simulink model "pid_pd_sim_2"  (R2016b)
settings: Solver=VariableStepAuto  StartTime=0.0  StopTime=100.0  FixedStep=1e-3  RelTol=1e3
values from neighbouring files (symbols this model uses):
  K_DG = part_vec(5)    [pso_tuning.m]
  K_filterG = 1/200    (= 0.005)    [pso_tuning.m]
undefined symbols (not defined in the file or in its folder): A_butter, B_butter, C_butter, D_butter, param, system
libraries: simulink x5
settings Model: Creator=nicol  LastModifiedBy=Fritz

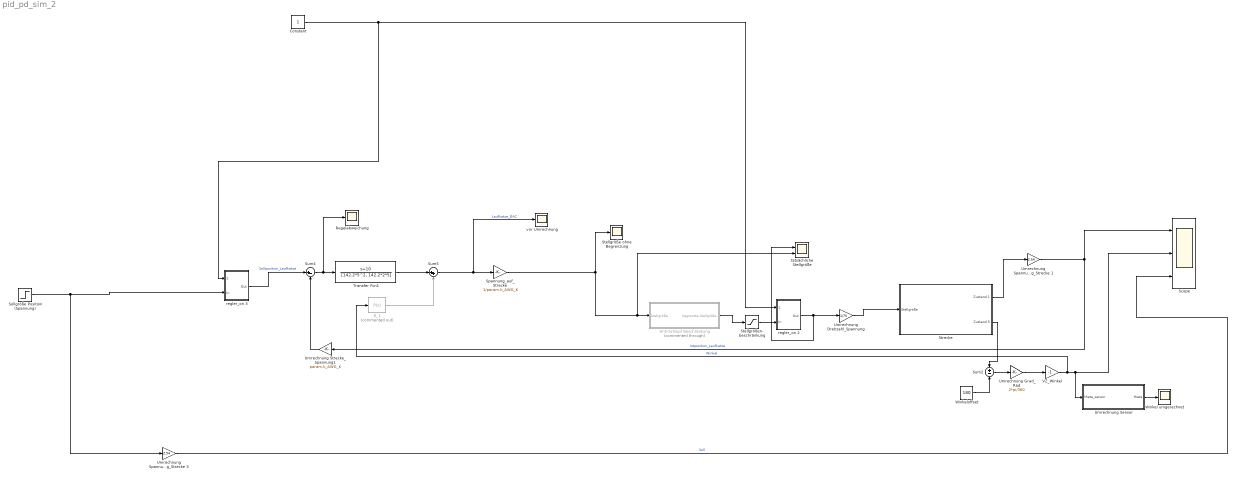
== system pid_pd_sim_2 ==
  Anti-Schlupf Beschränkung : Subsystem  Commented=through
  Constant : Constant
  R_1 : simulink/Continuous/PID Controller  Commented=on  Controller=P  TimeDomain=Continuous-time  SampleTime=-1  IntegratorMethod=Forward Euler  FilterMethod=Forward Euler  Form=Parallel  UseFilter=on  ControllerParametersSource=internal  P=0.1  I=0  D=K_DG  N=1/K_filterG  InitialConditionSource=internal  InitialConditionForIntegrator=0  InitialConditionForFilter=0  ExternalReset=none  LimitOutput=off  UpperSaturationLimit=inf  LowerSaturationLimit=-inf  LinearizeAsGain=on  AntiWindupMode=none  Kb=1  TrackingMode=off  Kt=1  PParamMin=[]  PParamMax=[]  IParamMin=[]  IParamMax=[]  DParamMin=[]  DParamMax=[]  NParamMin=[]  NParamMax=[]  KbParamMin=[]  KbParamMax=[]  KtParamMin=[]  KtParamMax=[]  POutMin=[]  POutMax=[]  IOutMin=[]  IOutMax=[]  DOutMin=[]  DOutMax=[]  NOutMin=[]  NOutMax=[]  KbOutMin=[]  KbOutMax=[]  KtOutMin=[]  KtOutMax=[]  IntegratorOutMin=[]  IntegratorOutMax=[]  FilterOutMin=[]  FilterOutMax=[]  SumOutMin=[]  SumOutMax=[]  SumI1OutMin=[]  SumI1OutMax=[]  SumI2OutMin=[]  SumI2OutMax=[]  SumI3OutMin=[]  SumI3OutMax=[]  SumDOutMin=[]  SumDOutMax=[]  SaturationOutMin=[]  SaturationOutMax=[]  IntegratorContinuousStateAttributes=''  IntegratorStateMustResolveToSignalObject=off  IntegratorRTWStateStorageClass=Auto  FilterContinuousStateAttributes=''  FilterStateMustResolveToSignalObject=off  FilterRTWStateStorageClass=Auto  DifferentiatorICPrevScaledInput=0  DifferentiatorOutMin=[]  DifferentiatorOutMax=[]
  Regelabweichung : Scope
  Scope : Scope  NumInputPorts=3
  Sollgröße Position (Spannung) : Step  Time=2  SampleTime=0
  Spannung_auf_Strecke : Gain  Gain=1/param.k_AWG_K
  Stellgröße ohne Begrenzung : Scope
  Stellgrößen- beschränkung : Saturate  UpperLimit=75  LowerLimit=-75
  Strecke : Subsystem
  Sum2 : Sum  Inputs=+|-
  Sum4 : Sum  Inputs=|+-
  Sum5 : Sum  Inputs=|++
  Transfer Fcn1 : TransferFcn  Numerator=[1 10]  Denominator=[142.2*5^2, 142.2*2*5]
  Umrechnung Drehzahl_Spannung : Gain  Gain=1/75
  Umrechnung Grad_Rad : Gain  Gain=2*pi/360
  Umrechnung Spannung_Strecke 1 : Gain  Gain=2.54
  Umrechnung Spannung_Strecke 3 : Gain  Gain=2.54
  Umrechnung Strecke_Spannung1 : Gain  Gain=param.k_AWG_K
  Umrechnung Sensor : MATLAB Function  TreatAsAtomicUnit=on
  VZ_Winkel : Gain  Gain=-1
  Winkel umgerechnet : Scope
  Winkeloffset : Constant  Value=180
  regler_on 2 : Subsystem
  regler_on 3 : Subsystem
  tatsächliche Stellgröße : Scope  NumInputPorts=2
  vor Umrechnung : Scope
  wires:
  Umrechnung Sensor/1(theta) -> Winkel umgerechnet/1
  Sum2/1 -> Umrechnung Grad_Rad/1
  Winkeloffset/1 -> Sum2/2
  Umrechnung Grad_Rad/1 -> VZ_Winkel/1
  Anti-Schlupf Beschränkung/1(begrenzte Stellgröße) -> Stellgrößen- beschränkung/1
  Sollgröße Position (Spannung)/1 -> regler_on 3/2(In), Umrechnung Spannung_Strecke 3/1
  Umrechnung Spannung_Strecke 3/1 -> Scope/3  "Soll"
  Constant/1 -> regler_on 3/1(regler_ on), regler_on 2/1(regler_ on)
  Strecke/2(Zustand 5) -> Sum2/1
  Strecke/1(Zustand 1) -> Umrechnung Spannung_Strecke 1/1
  Umrechnung Drehzahl_Spannung/1 -> Strecke/1(Stellgröße)
  regler_on 2/1(Out) -> Umrechnung Drehzahl_Spannung/1, tatsächliche Stellgröße/1
  Stellgrößen- beschränkung/1 -> regler_on 2/2(In)
  Sum5/1 -> vor Umrechnung/1, Spannung_auf_Strecke/1  "Laufkatze_DAC"
  R_1/1 -> Sum5/2
  VZ_Winkel/1 -> R_1/1, Umrechnung Sensor/1(theta_sensor), Scope/2  "Winkel"
  Transfer Fcn1/1 -> Sum5/1
  Sum4/1 -> Regelabweichung/1, Transfer Fcn1/1
  Umrechnung Spannung_Strecke 1/1 -> Scope/1, Umrechnung Strecke_Spannung1/1  "Istposition_Laufkatze"
  regler_on 3/1(Out) -> Sum4/1  "Sollposition_Laufkatze"
  Spannung_auf_Strecke/1 -> tatsächliche Stellgröße/2, Anti-Schlupf Beschränkung/1(Stellgröße), Stellgröße ohne Begrenzung/1
  Umrechnung Strecke_Spannung1/1 -> Sum4/2

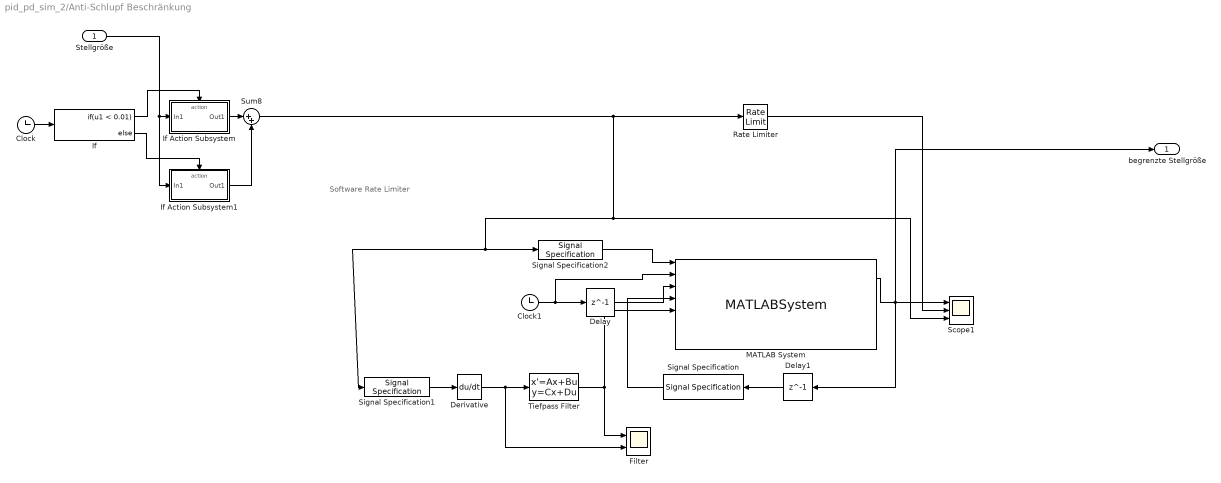
== system pid_pd_sim_2/Anti-Schlupf Beschränkung ==
  note: Software Rate Limiter
  Stellgröße : Inport
  Clock : Clock
  Clock1 : Clock
  Delay : Delay  DelayLength=1
  Delay1 : Delay  DelayLength=1
  Derivative : Derivative
  Filter : Scope  NumInputPorts=2
  If : If  IfExpression=u1 < 0.01
  If Action Subsystem : Subsystem  TreatAsAtomicUnit=on
  If Action Subsystem1 : Subsystem  TreatAsAtomicUnit=on
  MATLAB System : MATLABSystem  System=rate_limiter_classdef  SimulateUsing=Code generation
      mask Type: rate_limiter_classdef
      mask Display:
      | disp('rate_limiter_classdef');
      | port_label('input',1,'input');
      | port_label('input',2,'clock');
      | port_label('input',3,'clock_delayed');
      | port_label('input',4,'last_value');
      | port_label('input',5,'deriv');
      | port_label('input',6,'rate_limiter');
      | port_label('input',7,'rl_integral_in');
      | port_label('input',8,'rl_groesser_y_in');
      | port_label('output',1,'y');
      | port_label('output',2,'rl_integral_out');
      | port_label('output',3,'rl_groesser_y_out');
  Rate Limiter : RateLimiter  RisingSlewLimit=9.57  FallingSlewLimit=-9.57  SampleTimeMode=inherited
  Scope1 : Scope  NumInputPorts=3
  Signal Specification : SignalSpecification  OutDataTypeStr=double  Dimensions=1
  Signal Specification1 : SignalSpecification  Dimensions=1
  Signal Specification2 : SignalSpecification  Dimensions=1
  Sum8 : Sum  Inputs=|++
  Tiefpass Filter : StateSpace  A=A_butter  B=B_butter  C=C_butter  D=D_butter  X0=0
  begrenzte Stellgröße : Outport
  wires:
  Stellgröße/1 -> If Action Subsystem1/1(In1), If Action Subsystem/1(In1)
  If Action Subsystem/1(Out1) -> Sum8/1
  If Action Subsystem1/1(Out1) -> Sum8/2
  Clock/1 -> If/1
  If/1 -> If Action Subsystem/Action
  If/2 -> If Action Subsystem1/Action
  Sum8/1 -> Rate Limiter/1, Signal Specification1/1, Signal Specification2/1, Scope1/3
  Clock1/1 -> MATLAB System/2, Delay/1
  Delay/1 -> MATLAB System/3
  Delay1/1 -> Signal Specification/1
  Signal Specification/1 -> MATLAB System/4
  Signal Specification2/1 -> MATLAB System/1
  Signal Specification1/1 -> Derivative/1
  Derivative/1 -> Filter/2, Tiefpass Filter/1
  Tiefpass Filter/1 -> Filter/1, MATLAB System/5
  Rate Limiter/1 -> Scope1/2
  MATLAB System/1 -> begrenzte Stellgröße/1, Delay1/1, Scope1/1

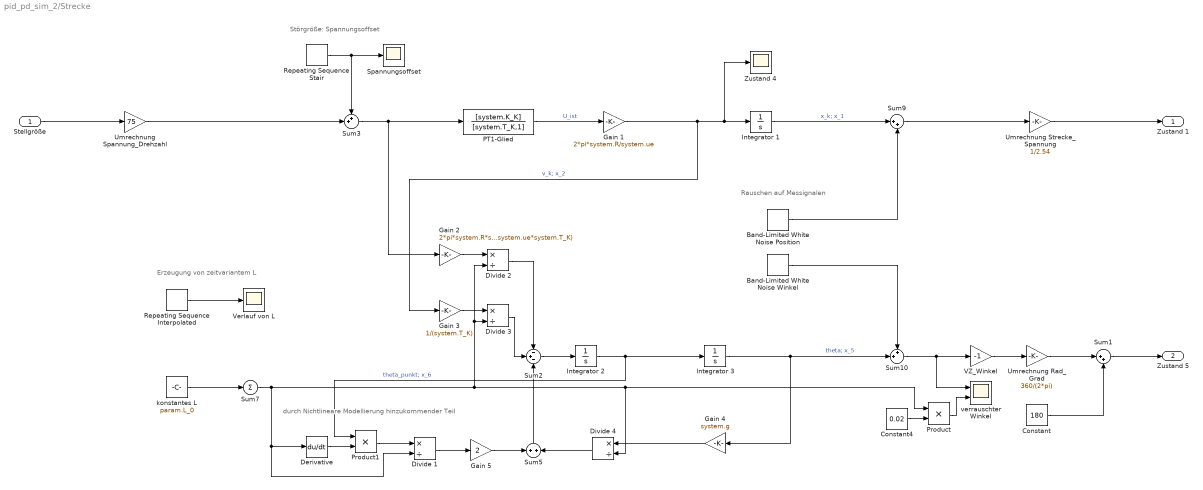
== system pid_pd_sim_2/Strecke ==
  note: Störgröße: Spannungsoffset
  note: durch Nichtlineare Modellierung hinzukommender Teil
  note: Rauschen auf Messignalen
  note: Erzeugung von zeitvariantem L
  Stellgröße : Inport
  Band-Limited White Noise Position : simulink/Sources/Band-Limited White Noise  Cov=[0.0000001]  Ts=0.01  seed=[23341]
  Band-Limited White Noise Winkel : simulink/Sources/Band-Limited White Noise  Cov=[0.000000001]  Ts=0.01  seed=[23341]
  Constant : Constant  Value=180
  Constant4 : Constant  Value=0.02
  Derivative : Derivative
  Divide {1..4} (4 alike) : Product  Inputs=*/
  Gain 1 : Gain  Gain=2*pi*system.R/system.ue
  Gain 2 : Gain  Gain=2*pi*system.R*system.K_K/(system.ue*system.T_K)
  Gain 3 : Gain  Gain=1/(system.T_K)
  Gain 4 : Gain  Gain=system.g
  Gain 5 : Gain  Gain=2
  Integrator 1 : Integrator
  Integrator 2 : Integrator
  Integrator 3 : Integrator
  PT1-Glied : TransferFcn  Numerator=[system.K_K]  Denominator=[system.T_K,1]
  Product : Product
  Product1 : Product
  Repeating Sequence Interpolated : simulink/Sources/Repeating Sequence Interpolated  OutValues=[1.5 1.0 0.7 0.5 0.4 0.3 0.2 0.5 1.5 1.0 0.2 0.2 1.0 1.5 0.5 0.2].'  TimeValues=[0 2 4 6 8 10 12 14 16 18 20 22 24 26 28 30].'  LookUpMeth=Interpolation-Use End Values  tsamp=0.001  OutMin=[]  OutMax=[]  OutDataTypeStr=double  OutputDataTypeScalingMode=double  OutDataType=fixdt(0,8)  OutScaling=2^-10
  Repeating Sequence Stair : simulink/Sources/Repeating Sequence Stair  OutValues=[0.02 0.05 0.05 0.02 0.08].'  tsamp=5  OutMin=[]  OutMax=[]  OutDataTypeStr=double  OutputDataTypeScalingMode=double  OutDataType=fixdt(0,8)  ConRadixGroup=Best Precision: Vector-wise  OutScaling=2^-12
  Spannungsoffset : Scope
  Sum1 : Sum  Inputs=|++
  Sum10 : Sum  Inputs=++|
  Sum2 : Sum  Inputs=-+-
  Sum3 : Sum  Inputs=++|
  Sum5 : Sum  Inputs=+|+
  Sum7 : Sum  Inputs=|+|
  Sum9 : Sum  Inputs=|++
  Umrechnung Rad_Grad : Gain  Gain=360/(2*pi)
  Umrechnung Spannung_Drehzahl : Gain  Gain=75
  Umrechnung Strecke_Spannung : Gain  Gain=1/2.54
  VZ_Winkel : Gain  Gain=-1
  Verlauf von L : Scope
  Zustand 4 : Scope
  konstantes L : Constant  Value=param.L_0
  verrauschter Winkel : Scope  NumInputPorts=2
  Zustand 1 : Outport
  Zustand 5 : Outport  Port=2
  wires:
  PT1-Glied/1 -> Gain 1/1  "U_ist"
  Gain 1/1 -> Zustand 4/1, Integrator 1/1, Gain 3/1  "v_k; x_2"
  Sum2/1 -> Integrator 2/1
  Integrator 2/1 -> Product1/1, Integrator 3/1  "theta_punkt; x_6"
  Integrator 3/1 -> Sum10/2, Gain 4/1  "theta; x_5"
  Sum3/1 -> PT1-Glied/1, Gain 2/1
  Repeating Sequence Stair/1 -> Sum3/1, Spannungsoffset/1
  Repeating Sequence Interpolated/1 -> Verlauf von L/1
  Gain 2/1 -> Divide 2/1
  Divide 2/1 -> Sum2/1
  Gain 3/1 -> Divide 3/1
  Divide 3/1 -> Sum2/2
  Gain 4/1 -> Divide 4/1
  Sum7/1 -> Divide 1/2, Derivative/1, Divide 3/2, Divide 2/2, Divide 4/2, Product/1
  Product/1 -> verrauschter Winkel/2
  Constant4/1 -> Product/2
  Integrator 1/1 -> Sum9/1  "x_k; x_1"
  Sum9/1 -> Umrechnung Strecke_Spannung/1
  Divide 4/1 -> Sum5/2
  Sum5/1 -> Sum2/3
  Gain 5/1 -> Sum5/1
  Product1/1 -> Divide 1/1
  Divide 1/1 -> Gain 5/1
  Derivative/1 -> Product1/2
  Stellgröße/1 -> Umrechnung Spannung_Drehzahl/1
  Umrechnung Spannung_Drehzahl/1 -> Sum3/2
  Umrechnung Strecke_Spannung/1 -> Zustand 1/1
  Sum10/1 -> VZ_Winkel/1, verrauschter Winkel/1
  Sum1/1 -> Zustand 5/1
  Umrechnung Rad_Grad/1 -> Sum1/1
  Constant/1 -> Sum1/2
  VZ_Winkel/1 -> Umrechnung Rad_Grad/1
  konstantes L/1 -> Sum7/1
  Band-Limited White Noise Position/1 -> Sum9/2
  Band-Limited White Noise Winkel/1 -> Sum10/1

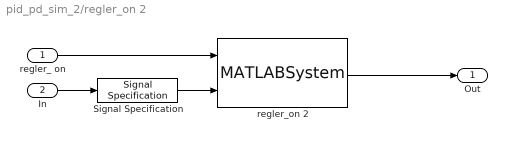
== system pid_pd_sim_2/regler_on 2 ==
  regler_ on : Inport
  In : Inport  Port=2
  Signal Specification : SignalSpecification  Dimensions=1
  regler_on 2 : MATLABSystem  System=regler_switch_1  SimulateUsing=Code generation
      mask Type: regler_switch_1
      mask Display:
      | disp('regler_switch_1');
      | port_label('input',1,'regler_on');
      | port_label('input',2,'input');
      | port_label('output',1,'y');
  Out : Outport
  wires:
  regler_ on/1 -> regler_on 2/1
  regler_on 2/1 -> Out/1
  Signal Specification/1 -> regler_on 2/2
  In/1 -> Signal Specification/1

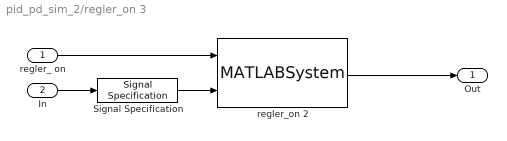
== system pid_pd_sim_2/regler_on 3 ==
  regler_ on : Inport
  In : Inport  Port=2
  Signal Specification : SignalSpecification  Dimensions=1
  regler_on 2 : MATLABSystem  System=regler_switch_1  SimulateUsing=Code generation
      mask Type: regler_switch_1
      mask Display:
      | disp('regler_switch_1');
      | port_label('input',1,'regler_on');
      | port_label('input',2,'input');
      | port_label('output',1,'y');
  Out : Outport
  wires:
  regler_ on/1 -> regler_on 2/1
  regler_on 2/1 -> Out/1
  Signal Specification/1 -> regler_on 2/2
  In/1 -> Signal Specification/1

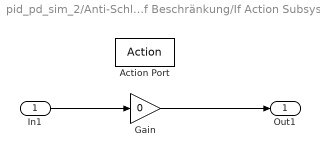
== system pid_pd_sim_2/Anti-Schlupf Beschränkung/If Action Subsystem ==
  In1 : Inport
  Action Port : ActionPort  ActionType=then
  Gain : Gain  Gain=0
  Out1 : Outport
  wires:
  In1/1 -> Gain/1
  Gain/1 -> Out1/1

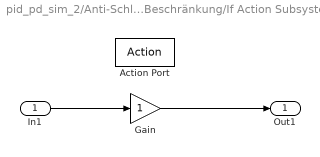
== system pid_pd_sim_2/Anti-Schlupf Beschränkung/If Action Subsystem1 ==
  In1 : Inport
  Action Port : ActionPort  ActionType=else
  Gain : Gain
  Out1 : Outport
  wires:
  In1/1 -> Gain/1
  Gain/1 -> Out1/1

== matlab function pid_pd_sim_2/Umrechnung Sensor ==
  data: theta_sensor input; theta output
function theta  = sensorWinkel(theta_sensor)
% berechnet aus dem gemessenen Winkel den tatsächlichen Winkel des
% Lasthebers

% l_verb: Länge des Verbindungsstücks
% l_welle: Abstand der beiden Wellen

% Parameter für die Winkelumrechnung
l_verb = 0.109; % m %
l_welle = 0.0575; % m %

theta = asin(sin(theta_sensor) * (l_verb / sqrt(l_welle^2 + l_verb^2 - (2 * l_verb * l_welle * cos(theta_sensor)))));
